simulink library "ddm"  (R2021b)
settings: Solver=VariableStepAuto  StartTime=0.0  StopTime=10.0  RelTol=1e-3
undefined symbols (not defined in the file or in its folder): ADDM_FrTMTqDev_X_Nm, ADDM_RrTMTqDev_X_Nm, ENUM_ADASACCSTA_ERROR, ENUM_ADASACCSTA_OFF, ENUM_ADASACCSTA_STANDBY, ENUM_ALLOWMOV_ALLOWREADY, ENUM_APS, ENUM_BRKSTA_ERROR, ENUM_BRKSTA_OFF, ENUM_BRKSTA_ON, ENUM_BRKSW_INVALID, ENUM_BRKSW_OFF, ENUM_BRKSW_ON, ENUM_CHGPREACTERRSTA_OBCPRE, ENUM_DCDCFAULTSTA_ANYFAULTLV1, ENUM_DCDCFAULTSTA_ANYFAULTLV2, ENUM_DRIVETRAIN_AWD, ENUM_DRIVETRAIN_FWD, ENUM_DRIVETRAIN_RWD, ENUM_EDUDRTSTA_NORMAL, ENUM_EPBSTA_APPLIED, ENUM_EPBSTA_RELEASED, ENUM_GEARACTUALPOSN_INVALID, ENUM_GEARACTUALPOSN_P, ENUM_HVBATTREADYPRE_READY, ENUM_MCUWARN_LV0, ENUM_MCUWARN_LV1, ENUM_MCUWARN_LV2, ENUM_MCUWARN_LV3, ENUM_MCUWARN_NOERROR, ENUM_OBCFAULTSTA_ANYFAULT, ENUM_PAS_R2F2, ENUM_PDFAULT_BATTPDFAIL, ENUM_PDFAULT_DCDCDISABLE, ENUM_PDFAULT_MCUDISABLE, ENUM_PDFAULT_MCUDISCHRG, ENUM_POWERSTA_OFF, ENUM_POWERSTA_ON, ENUM_POWERSTA_READY, ENUM_POWERSTA_STANDBY, ENUM_PRESSINDI_LOW, ENUM_PUFAULT_BATTUPFAIL, ENUM_PUFAULT_DCDCENABLEFAIL, ENUM_PUFAULT_PRECHRGCHKFAIL, ENUM_PUFAULT_SAFETYCHKFAIL, ENUM_PUSTATE_COMPLETED, ENUM_PWRSTASW_OFF, ENUM_PWRSTASW_OFFA, ENUM_PWRSTASW_OFFCHVCHRG, ENUM_PWRSTASW_OFFCLVCHRG, ENUM_PWRSTASW_ON, ENUM_PWRSTASW_ONHVCHRG, ENUM_PWRSTASW_READY, ENUM_PWRSTASW_STANDBY, ENUM_SHIFTCOMMAND_P, ENUM_SHIFTERERRSTA_PBUTTONFAILURE, ENUM_VEHMALFUNLV_2ND, ENUM_VEHMALFUNLV_3RD, ENUM_VEHMALFUNLV_4TH, ENUM_VEHMALFUNLV_NORMAL ... (+459)
libraries: hcu_lib x521, $bdroot x5, simulink x3
(part 14 of 25)

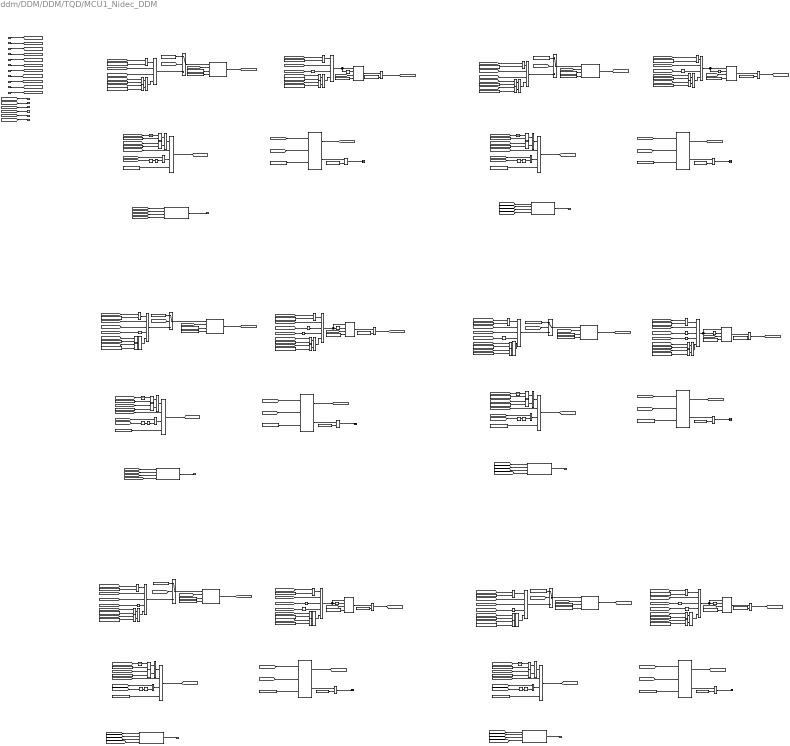
== system ddm/DDM/DDM/TQD/MCU1_Nidec_DDM ==
  note: Diagnostics and Fault Handling
  note: Release Condition After Decision
  note: Diagnostics and Fault Handling
  note: Release Condition After Decision
  note: Diagnostics and Fault Handling
  note: Release Condition After Decision
  note: Release Condition After Decision
  note: Diagnostics and Fault Handling
  note: Release Condition After Decision
  note: Diagnostics and Fault Handling
  note: Release Condition After Decision
  note: Diagnostics and Fault Handling
  note: MCU_F1 Lost Comm (MCUF1NoCom)
  note: MCU_R1 Lost Comm (MCUR1NoCom)
  note: MCU_R1 Rolling Count Error (MCUR1RCErr)
  note: MCU_F1 Rolling Count Error (MCUF1RCErr)
  note: MCU_R1 Checksum Error (MCUR1CSErr)
  note: MCU_F1 Checksum Error (MCUF1CSErr)
  task_time_s : Inport
  VPMM_SysPwrSta_enum : Inport  Port=2
  No_CAN3_BUS_OFF : Inport  Port=3
  VDDM_MCUNF1NoCom_flg : Inport  Port=4
  VDDM_MCUNR1NoCom_flg : Inport  Port=5
  VDDM_MCUNF1RCErr_flg : Inport  Port=6
  VDDM_MCUNF1CSErr_flg : Inport  Port=7
  VDDM_MCUNR1RCErr_flg : Inport  Port=8
  VDDM_MCUNR1CSErr_flg : Inport  Port=9
  DTC_clear_request : Inport  Port=10
  VPMM_DrivetrainSelect_enum : Inport  Port=11
  Constant{1..2,6..7,9,13,26,40,43,46,53,59..60,62,72,75,79,86} (18 alike) : Constant  Value=ENUM_PWRSTASW_OFF
  Constant{3,10,35,41,52,57} (6 alike) : Constant  Value=ENUM_PWRSTASW_STANDBY
  Constant{20,24,28,44,67,88,90,92,94,96,98,100} (12 alike) : Constant  Value=ENUM_DRIVETRAIN_AWD
  Constant{4,11,29,45,55,101} (6 alike) : Constant  Value=KDDM_TQDDiagnosisOffSW_flg
  Constant{5,12,30,49,56,102} (6 alike) : Constant  Value=ZERO_INT
  Constant14 : Constant  Value=KDDM_MCUF1NoComDTC_cnt
  Constant{15,27,66,93,95,97} (6 alike) : Constant  Value=ENUM_DRIVETRAIN_RWD
  Constant16 : Constant  Value=KDDM_MCUNR1NoComDTC_cnt
  Constant17 : Constant  Value=KDDM_MCUNR1NoComPassTO_s
  Constant18 : Constant  Value=KDDM_MCUNR1NoComPassTO_s
  Constant19 : Constant  Value=KDDM_MCUNR1NoComDetTO_s
  Constant{21,42,87,89,91,99} (6 alike) : Constant  Value=ENUM_DRIVETRAIN_FWD
  Constant{22..23,38..39,73..74} (6 alike) : Constant  Value=FALSE
  Constant25 : Constant  Value=KDDM_MCUF1RCErrDTC_cnt
  Constant31 : Constant  Value=KDDM_MCUNR1RCErrDTC_cnt
  Constant32 : Constant  Value=KDDM_MCUNR1RCErrPassTO_s
  Constant33 : Constant  Value=KDDM_MCUNR1RCErrPassTO_s
  Constant34 : Constant  Value=KDDM_MCUNR1RCErrDetTO_s
  Constant36 : Constant  Value=KDDM_MCUR1RCErrDTC_cnt
  Constant37 : Constant  Value=KDDM_MCUNF1CSErrPassTO_s
  Constant47 : Constant  Value=KDDM_MCUNF1RCErrDTC_cnt
  Constant48 : Constant  Value=KDDM_MCUNF1RCErrPassTO_s
  Constant50 : Constant  Value=KDDM_MCUNF1RCErrPassTO_s
  Constant51 : Constant  Value=KDDM_MCUNF1RCErrDetTO_s
  Constant54 : Constant  Value=KDDM_MCUF1RCErrDTC_cnt
  Constant58 : Constant  Value=KDDM_MCUR1RCErrDTC_cnt
  Constant61 : Constant  Value=KDDM_MCUNR1CSErrDTC_cnt
  Constant63 : Constant  Value=KDDM_MCUNR1CSErrPassTO_s
  Constant64 : Constant  Value=KDDM_MCUNR1CSErrPassTO_s
  Constant65 : Constant  Value=KDDM_MCUNR1CSErrDetTO_s
  Constant68 : Constant  Value=KDDM_MCUNF1NoComDTC_cnt
  Constant69 : Constant  Value=KDDM_MCUNF1NoComPassTO_s
  Constant70 : Constant  Value=KDDM_MCUNF1NoComPassTO_s
  Constant71 : Constant  Value=KDDM_MCUNF1NoComDetTO_s
  Constant8 : Constant  Value=KDDM_MCUR1NoComDTC_cnt
  Constant80 : Constant  Value=KDDM_MCUNF1CSErrDTC_cnt
  Constant83 : Constant  Value=KDDM_MCUNF1CSErrPassTO_s
  Constant84 : Constant  Value=KDDM_MCUNF1CSErrDetTO_s
  DTC_Couter{1..5,7} (6 alike) : hcu_lib/Basic_Blocks/DTC_Couter
  DTC_Info{,1..5} (6 alike) : hcu_lib/Basic_Blocks/DTC_Info
  Delay{1..6} (6 alike) : Delay  DelayLength=1
  Equal{,1..4,7..8,12,14..15,19..20,23,26..27,33..43,45,47..55} (36 alike) : RelationalOperator  Operator===  OutDataTypeStr=boolean  RndMeth=Simplest
  Equal{5,9..11,16,18,21..22,24,29,44,46} (12 alike) : RelationalOperator  Operator=~=  OutDataTypeStr=boolean  RndMeth=Simplest
  Equal{6,13,17,25,28,30} (6 alike) : RelationalOperator  OutDataTypeStr=boolean  RndMeth=Simplest
  Logical Operator{1,3,16,21,33,36} (6 alike) : Logic  Operator=OR  Inputs=4  AllPortsSameDT=off  OutDataTypeStr=boolean
  Logical Operator{6,10,13,15,19..20,24..26,29,32,37,41..42,61,70,81..84} (20 alike) : Logic  Operator=NOT  AllPortsSameDT=off  OutDataTypeStr=boolean
  Logical Operator{4,8..9,11,17..18,22,28,34..35,38..39} (12 alike) : Logic  AllPortsSameDT=off  OutDataTypeStr=boolean
  Logical Operator{7,12,23,27,31,40,58,67} (8 alike) : Logic  Inputs=5  AllPortsSameDT=off  OutDataTypeStr=boolean
  Logical Operator{2,5,14,30} (4 alike) : Logic  Inputs=4  AllPortsSameDT=off  OutDataTypeStr=boolean
  NOT{1..6} (6 alike) : Logic  Operator=NOT  AllPortsSameDT=off  OutDataTypeStr=boolean
  OR{,1..11} (12 alike) : Logic  Operator=OR  AllPortsSameDT=off  OutDataTypeStr=boolean
  Relational Operator{1..6} (6 alike) : RelationalOperator  Operator=>  OutDataTypeStr=boolean  RndMeth=Simplest
  Switch{1..6} (6 alike) : Switch  Criteria=u2 ~= 0
  Terminator{,1..5} (6 alike) : Terminator
  Test Detection Criteria{1..6} (6 alike) : hcu_lib/Basic_Blocks/Test Detection Criteria
  Timer{1..6} (6 alike) : hcu_lib/Basic_Blocks/Timer
  Unit Delay{1..4,6..7} (6 alike) : UnitDelay  SampleTime=-1  HasFrameUpgradeWarning=on
  VDDM_MCUF1NoComDTC_raw32 : Outport
  VDDM_MCUR1NoComDTC_raw32 : Outport  Port=2
  VDDM_MCUF1RCErrDTC_raw32 : Outport  Port=3
  VDDM_MCUR1RCErrDTC_raw32 : Outport  Port=4
  VDDM_MCUF1CSErrDTC_raw32 : Outport  Port=5
  VDDM_MCUR1CSErrDTC_raw32 : Outport  Port=6
  VDDM_MCUNF1NoComCFS_flg : Outport  Port=7
  VDDM_MCUNF1RCErrCFS_flg : Outport  Port=8
  VDDM_MCUNF1CSErrCFS_flg : Outport  Port=9
  VDDM_MCUNR1NoComCFS_flg : Outport  Port=10
  VDDM_MCUNR1RCErrCFS_flg : Outport  Port=11
  VDDM_MCUNR1CSErrCFS_flg : Outport  Port=12
  wires:
  Logical Operator42/1 -> Logical Operator40/3
  [VDDM_MCUNR1CSErr_flg] -> Logical Operator42/1
  [VPMM_DrivetrainSelect_enum] -> Equal54/1
  Logical Operator41/1 -> Logical Operator40/4
  Constant67/1 -> Equal55/2
  [VPMM_DrivetrainSelect_enum] -> Equal55/1
  Equal22/1 -> Logical Operator40/1
  Constant66/1 -> Equal54/2
  OR11/1 -> Logical Operator40/5
  Equal55/1 -> OR11/2
  [No_CAN3_BUS_OFF] -> Logical Operator40/2
  Constant60/1 -> Equal22/2
  [VDDM_MCUNR1NoComCFS_flg] -> Logical Operator41/1
  Equal54/1 -> OR11/1
  [VPMM_SysPwrSta_enum] -> Equal22/1
  [VPMM_SysPwrSta_enum] -> Unit Delay4/1
  NOT6/1 -> Logical Operator39/2
  [VDDM_MCUNR1CSErrPass_flg] -> Logical Operator39/1
  DTC_Couter5/2 -> Relational Operator6/1  "VDDM_MCUNR1CSErrDTC_cnt"
  Constant59/1 -> Equal27/2
  Relational Operator6/1 -> Terminator5/1  "VDDM_MCUNR1CSErrDFS_flg"
  Delay6/1 -> NOT6/1
  Unit Delay4/1 -> Equal27/1
  Constant58/1 -> DTC_Couter5/3
  Equal26/1 -> Logical Operator38/2
  Equal27/1 -> Logical Operator38/1
  [VPMM_SysPwrSta_enum] -> Equal26/1
  Logical Operator39/1 -> Logical Operator36/3
  Constant55/1 -> Logical Operator36/4
  Constant57/1 -> Equal26/2
  Logical Operator38/1 -> Logical Operator36/1
  Logical Operator36/1 -> [VDDM_MCUNR1CSErrCFSRls_flg]  "VDDM_MCUNR1CSErrCFSRls_flg"
  Constant56/1 -> Relational Operator6/2
  [VDDM_MCUNR1CSErrDet_flg] -> DTC_Couter5/1
  [DTC_clear_request] -> Logical Operator36/2
  [VDDM_MCUNR1CSErrCFS_flg] -> Delay6/1
  DTC_Couter5/1 -> [VDDM_MCUNR1CSErrCFS_flg]  "VDDM_MCUNR1CSErrCFS_flg"
  [VDDM_MCUNR1CSErrCFSRls_flg] -> DTC_Couter5/2
  [VPMM_SysPwrSta_enum] -> Equal52/1
  Constant75/1 -> Equal53/2
  [VDDM_MCUNF1CSErrDet_flg] -> DTC_Couter4/1
  Delay5/1 -> NOT5/1
  Unit Delay3/1 -> Equal53/1
  [VDDM_MCUNF1CSErrCFSRls_flg] -> DTC_Couter4/2
  Constant54/1 -> DTC_Couter4/3
  Equal53/1 -> Logical Operator34/1
  Equal52/1 -> Logical Operator34/2
  [VPMM_SysPwrSta_enum] -> Unit Delay3/1
  NOT5/1 -> Logical Operator35/2
  Logical Operator34/1 -> Logical Operator33/1
  Constant52/1 -> Equal52/2
  Constant45/1 -> Logical Operator33/4
  [DTC_clear_request] -> Logical Operator33/2
  Logical Operator35/1 -> Logical Operator33/3
  DTC_Couter4/2 -> Relational Operator5/1  "VDDM_MCUNF1CSErrDTC_cnt"
  [VDDM_MCUNF1CSErrPass_flg] -> Logical Operator35/1
  Logical Operator33/1 -> [VDDM_MCUNF1CSErrCFSRls_flg]  "VDDM_MCUNF1CSErrCFSRls_flg"
  Constant49/1 -> Relational Operator5/2
  Relational Operator5/1 -> Terminator4/1  "VDDM_MCUNF1CSErrDFS_flg"
  DTC_Couter4/1 -> [VDDM_MCUNF1CSErrCFS_flg]  "VDDM_MCUNF1CSErrCFS_flg"
  [VDDM_MCUNF1CSErrCFS_flg] -> Delay5/1
  Logical Operator32/1 -> Logical Operator27/3
  OR10/1 -> Logical Operator27/5
  Equal20/1 -> OR10/2
  Equal19/1 -> OR10/1
  [VPMM_DrivetrainSelect_enum] -> Equal19/1
  Constant42/1 -> Equal19/2
  Constant44/1 -> Equal20/2
  [VPMM_DrivetrainSelect_enum] -> Equal20/1
  [VDDM_MCUNF1NoComCFS_flg] -> Logical Operator29/1
  Logical Operator29/1 -> Logical Operator27/4
  [VDDM_MCUNF1CSErr_flg] -> Logical Operator32/1
  Constant40/1 -> Equal18/2
  Equal18/1 -> Logical Operator27/1
  [No_CAN3_BUS_OFF] -> Logical Operator27/2
  [VPMM_SysPwrSta_enum] -> Equal18/1
  Logical Operator6/1 -> Logical Operator5/3
  Logical Operator25/1 -> Timer2/2
  Logical Operator24/1 -> Logical Operator2/3
  Logical Operator10/1 -> Timer1/2
  [VPMM_SysPwrSta_enum] -> Equal15/1
  Constant43/1 -> Equal51/2
  [VDDM_MCUNR1RCErrDet_flg] -> DTC_Couter3/1
  Delay4/1 -> NOT4/1
  Unit Delay2/1 -> Equal51/1
  [VDDM_MCUNR1RCErrCFSRls_flg] -> DTC_Couter3/2
  Constant36/1 -> DTC_Couter3/3
  Equal51/1 -> Logical Operator22/1
  Equal15/1 -> Logical Operator22/2
  [VPMM_SysPwrSta_enum] -> Unit Delay2/1
  NOT4/1 -> Logical Operator28/2
  Logical Operator22/1 -> Logical Operator21/1
  Constant35/1 -> Equal15/2
  Constant29/1 -> Logical Operator21/4
  [DTC_clear_request] -> Logical Operator21/2
  Logical Operator28/1 -> Logical Operator21/3
  DTC_Couter3/2 -> Relational Operator4/1  "VDDM_MCUNR1RCErrDTC_cnt"
  [VDDM_MCUNR1RCErrPass_flg] -> Logical Operator28/1
  Logical Operator21/1 -> [VDDM_MCUNR1RCErrCFSRls_flg]  "VDDM_MCUNR1RCErrCFSRls_flg"
  Constant30/1 -> Relational Operator4/2
  Relational Operator4/1 -> Terminator3/1  "VDDM_MCUNR1RCErrDFS_flg"
  DTC_Couter3/1 -> [VDDM_MCUNR1RCErrCFS_flg]  "VDDM_MCUNR1RCErrCFS_flg"
  [VDDM_MCUNR1RCErrCFS_flg] -> Delay4/1
  Logical Operator20/1 -> Logical Operator7/3
  OR9/1 -> Logical Operator7/5
  [VPMM_DrivetrainSelect_enum] -> Equal14/1
  Constant27/1 -> Equal12/2
  Equal14/1 -> OR9/2
  [VPMM_DrivetrainSelect_enum] -> Equal12/1
  Constant28/1 -> Equal14/2
  Equal12/1 -> OR9/1
  [VDDM_MCUNR1NoComCFS_flg] -> Logical Operator19/1
  Logical Operator19/1 -> Logical Operator7/4
  [No_CAN3_BUS_OFF] -> Logical Operator7/2
  Equal10/1 -> Logical Operator7/1
  Constant26/1 -> Equal10/2
  [VDDM_MCUNR1RCErr_flg] -> Logical Operator20/1
  [VPMM_SysPwrSta_enum] -> Equal10/1
  Delay3/1 -> NOT3/1
  [VDDM_MCUNF1RCErrCFS_flg] -> Delay3/1
  Constant101/1 -> Logical Operator16/4
  [DTC_clear_request] -> Logical Operator16/2
  NOT3/1 -> Logical Operator18/2
  Constant41/1 -> Equal49/2
  Logical Operator17/1 -> Logical Operator16/1
  [VPMM_SysPwrSta_enum] -> Unit Delay7/1
  Relational Operator3/1 -> Terminator2/1  "VDDM_MCUNF1RCErrDFS_flg"
  Equal49/1 -> Logical Operator17/2
  Constant72/1 -> Equal50/2
  Unit Delay7/1 -> Equal50/1
  [VPMM_SysPwrSta_enum] -> Equal49/1
  Equal50/1 -> Logical Operator17/1
  [VDDM_MCUNF1RCErrPass_flg] -> Logical Operator18/1
  Logical Operator18/1 -> Logical Operator16/3
  Constant25/1 -> DTC_Couter7/3
  DTC_Couter7/1 -> [VDDM_MCUNF1RCErrCFS_flg]  "VDDM_MCUNF1RCErrCFS_flg"
  Logical Operator16/1 -> [VDDM_MCUNF1RCErrCFSRls_flg]  "VDDM_MCUNF1RCErrCFSRls_flg"
  [VDDM_MCUNF1RCErrCFSRls_flg] -> DTC_Couter7/2
  DTC_Couter7/2 -> Relational Operator3/1  "VDDM_MCUNF1RCErrDTC_cnt"
  [VDDM_MCUNF1RCErrDet_flg] -> DTC_Couter7/1
  Constant102/1 -> Relational Operator3/2
  Logical Operator15/1 -> Logical Operator12/3
  [VPMM_DrivetrainSelect_enum] -> Equal48/1
  Constant24/1 -> Equal48/2
  [VDDM_MCUNF1NoComCFS_flg] -> Logical Operator13/1
  Equal47/1 -> OR8/1
  [VPMM_SysPwrSta_enum] -> Equal9/1
  Logical Operator13/1 -> Logical Operator12/4
  Constant21/1 -> Equal47/2
  Equal9/1 -> Logical Operator12/1
  Equal48/1 -> OR8/2
  [VPMM_DrivetrainSelect_enum] -> Equal47/1
  OR8/1 -> Logical Operator12/5
  [VDDM_MCUNF1RCErr_flg] -> Logical Operator15/1
  Constant7/1 -> Equal9/2
  [No_CAN3_BUS_OFF] -> Logical Operator12/2
  Delay2/1 -> NOT2/1
  [VDDM_MCUNR1NoComCFS_flg] -> Delay2/1
  Constant4/1 -> Logical Operator1/4
  [DTC_clear_request] -> Logical Operator1/2
  NOT2/1 -> Logical Operator11/2
  Constant3/1 -> Equal7/2
  Logical Operator9/1 -> Logical Operator1/1
  [VPMM_SysPwrSta_enum] -> Unit Delay1/1
  Relational Operator1/1 -> Terminator1/1  "VDDM_MCUNR1NoComDFS_flg"
  Equal7/1 -> Logical Operator9/2
  Constant6/1 -> Equal8/2
  Unit Delay1/1 -> Equal8/1
  [VPMM_SysPwrSta_enum] -> Equal7/1
  Equal8/1 -> Logical Operator9/1
  [VDDM_MCUNR1NoComPass_flg] -> Logical Operator11/1
  Logical Operator11/1 -> Logical Operator1/3
  Constant8/1 -> DTC_Couter2/3
  DTC_Couter2/1 -> [VDDM_MCUNR1NoComCFS_flg]  "VDDM_MCUNR1NoComCFS_flg"
  Logical Operator1/1 -> [VDDM_MCUNR1NoComCFSRls_flg]  "VDDM_MCUNR1NoComCFSRls_flg"
  [VDDM_MCUNR1NoComCFSRls_flg] -> DTC_Couter2/2
  DTC_Couter2/2 -> Relational Operator1/1  "VDDM_MCUNR1NoComDTC_cnt"
  [VDDM_MCUNR1NoComDet_flg] -> DTC_Couter2/1
  Constant5/1 -> Relational Operator1/2
  Logical Operator5/1 -> Logical Operator25/1, Timer2/1
  Equal2/1 -> OR7/1
  Constant20/1 -> Equal23/2
  OR7/1 -> Logical Operator5/4
  [VPMM_DrivetrainSelect_enum] -> Equal2/1
  Equal23/1 -> OR7/2
  Constant15/1 -> Equal2/2
  [VPMM_DrivetrainSelect_enum] -> Equal23/1
  [No_CAN3_BUS_OFF] -> Logical Operator5/2
  Constant2/1 -> Equal46/2
  [VDDM_MCUNR1NoCom_flg] -> Logical Operator6/1
  Equal46/1 -> Logical Operator5/1
  [VPMM_SysPwrSta_enum] -> Equal46/1
  Constant13/1 -> Equal4/2
  [VPMM_SysPwrSta_enum] -> Equal3/1
  Constant10/1 -> Equal3/2
  Equal4/1 -> Logical Operator4/1
  [DTC_clear_request] -> Logical Operator3/2
  Logical Operator8/1 -> Logical Operator3/3
  Logical Operator4/1 -> Logical Operator3/1
  [VDDM_MCUNF1NoComPass_flg] -> Logical Operator8/1
  Constant11/1 -> Logical Operator3/4
  Logical Operator3/1 -> [VDDM_MCUNF1NoComCFSRls_flg]  "VDDM_MCUNF1NoComCFSRls_flg"
  NOT1/1 -> Logical Operator8/2
  [VDDM_MCUNF1NoComCFS_flg] -> Delay1/1
  Delay1/1 -> NOT1/1
  Equal3/1 -> Logical Operator4/2
  Unit Delay6/1 -> Equal4/1
  [VPMM_SysPwrSta_enum] -> Unit Delay6/1
  DTC_Couter1/2 -> Relational Operator2/1  "VDDM_MCUNF1NoComDTC_cnt"
  Relational Operator2/1 -> Terminator/1  "VDDM_MCUNF1NoComDFS_flg"
  Constant12/1 -> Relational Operator2/2
  Logical Operator2/1 -> Logical Operator10/1, Timer1/1
  [VPMM_SysPwrSta_enum] -> Equal44/1
  Equal1/1 -> OR6/1
  [VDDM_MCUNF1NoCom_flg] -> Logical Operator24/1
  Constant99/1 -> Equal1/2
  Equal44/1 -> Logical Operator2/1
  Constant100/1 -> Equal45/2
  [No_CAN3_BUS_OFF] -> Logical Operator2/2
  [VPMM_DrivetrainSelect_enum] -> Equal45/1
  OR6/1 -> Logical Operator2/4
  Equal45/1 -> OR6/2
  Constant1/1 -> Equal44/2
  [VPMM_DrivetrainSelect_enum] -> Equal1/1
  [VDDM_MCUNF1NoCom_flg] -> Logical Operator30/3
  Equal21/1 -> Logical Operator30/1
  [No_CAN3_BUS_OFF] -> Logical Operator30/2
  Timer1/1 -> Equal28/1
  [VDDM_MCUNF1NoComDet_flg] -> DTC_Couter1/1
  [VPMM_SysPwrSta_enum] -> Equal21/1
  Constant70/1 -> Timer1/4
  [task_time_s] -> Timer1/3
  Test Detection Criteria1/1 -> [VDDM_MCUNF1NoComDet_flg]  "VDDM_MCUNF1NoComDet_flg"
  Constant62/1 -> Equal21/2
  Constant69/1 -> Equal28/2
  Equal28/1 -> [VDDM_MCUNF1NoComPass_flg]  "VDDM_MCUNF1NoComPass_flg"
  [task_time_s] -> Test Detection Criteria1/2
  Constant68/1 -> Test Detection Criteria1/3
  Constant71/1 -> Test Detection Criteria1/4
  Constant14/1 -> DTC_Couter1/3
  [VDDM_MCUNF1NoComCFSRls_flg] -> DTC_Couter1/2
  [VPMM_SysPwrSta_enum] -> Equal5/1
  Equal5/1 -> Logical Operator14/1
  Constant19/1 -> Test Detection Criteria2/4
  Timer2/1 -> Equal6/1
  Equal6/1 -> [VDDM_MCUNR1NoComPass_flg]  "VDDM_MCUNR1NoComPass_flg"
  Test Detection Criteria2/1 -> [VDDM_MCUNR1NoComDet_flg]  "VDDM_MCUNR1NoComDet_flg"
  Constant16/1 -> Test Detection Criteria2/3
  [VDDM_MCUNR1NoCom_flg] -> Logical Operator14/3
  Constant18/1 -> Timer2/4
  Constant9/1 -> Equal5/2
  [No_CAN3_BUS_OFF] -> Logical Operator14/2
  [task_time_s] -> Test Detection Criteria2/2
  Constant17/1 -> Equal6/2
  [task_time_s] -> Timer2/3
  [VDDM_MCUNF1NoComCFS_flg] -> DTC_Info/3
  [VDDM_MCUNF1NoComPass_flg] -> DTC_Info/2
  [VDDM_MCUNF1NoComDet_flg] -> DTC_Info/1
  DTC_Info/1 -> VDDM_MCUF1NoComDTC_raw32/1  "VDDM_MCUF1NoComDTC_raw32"
  [VDDM_MCUNR1NoComDet_flg] -> DTC_Info1/1
  DTC_Info1/1 -> VDDM_MCUR1NoComDTC_raw32/1  "VDDM_MCUR1NoComDTC_raw32"
  [VDDM_MCUNR1NoComCFS_flg] -> DTC_Info1/3
  [VDDM_MCUNR1NoComPass_flg] -> DTC_Info1/2
  task_time_s/1 -> [task_time_s]
  VPMM_SysPwrSta_enum/1 -> [VPMM_SysPwrSta_enum]
  No_CAN3_BUS_OFF/1 -> [No_CAN3_BUS_OFF]
  VDDM_MCUNF1NoCom_flg/1 -> [VDDM_MCUNF1NoCom_flg]
  DTC_clear_request/1 -> [DTC_clear_request]
  VDDM_MCUNR1NoCom_flg/1 -> [VDDM_MCUNR1NoCom_flg]
  DTC_Couter1/1 -> [VDDM_MCUNF1NoComCFS_flg]  "VDDM_MCUNF1NoComCFS_flg"
  [DTC_clear_request] -> DTC_Info/4
  [DTC_clear_request] -> DTC_Info1/4
  [VDDM_MCUNF1NoComCFSRls_flg] -> Switch6/2
  Switch6/1 -> Test Detection Criteria1/1
  Constant22/1 -> Switch6/1
  Logical Operator30/1 -> Switch6/3
  [VDDM_MCUNR1NoComCFSRls_flg] -> Switch1/2
  Switch1/1 -> Test Detection Criteria2/1
  Constant23/1 -> Switch1/1
  [VPMM_SysPwrSta_enum] -> Equal11/1
  [No_CAN3_BUS_OFF] -> Logical Operator31/2
  Logical Operator37/1 -> Timer3/2
  [VPMM_SysPwrSta_enum] -> Equal16/1
  Timer3/1 -> Equal13/1
  Constant48/1 -> Equal13/2
  Logical Operator7/1 -> Timer4/1, Logical Operator26/1
  Test Detection Criteria3/1 -> [VDDM_MCUNF1RCErrDet_flg]  "VDDM_MCUNF1RCErrDet_flg"
  Constant51/1 -> Test Detection Criteria3/4
  Equal11/1 -> Logical Operator31/1
  Constant50/1 -> Timer3/4
  Constant34/1 -> Test Detection Criteria4/4
  Constant46/1 -> Equal11/2
  Equal17/1 -> [VDDM_MCUNR1RCErrPass_flg]  "VDDM_MCUNR1RCErrPass_flg"
  [VDDM_MCUNF1RCErr_flg] -> Logical Operator31/3
  Test Detection Criteria4/1 -> [VDDM_MCUNR1RCErrDet_flg]  "VDDM_MCUNR1RCErrDet_flg"
  DTC_Info2/1 -> VDDM_MCUF1RCErrDTC_raw32/1  "VDDM_MCUF1RCErrDTC_raw32"
  [VDDM_MCUNF1RCErrDet_flg] -> DTC_Info2/1
  [VDDM_MCUNF1RCErrPass_flg] -> DTC_Info2/2
  DTC_Info3/1 -> VDDM_MCUR1RCErrDTC_raw32/1  "VDDM_MCUR1RCErrDTC_raw32"
  [task_time_s] -> Timer4/3
  [task_time_s] -> Test Detection Criteria3/2
  [VDDM_MCUNR1RCErrPass_flg] -> DTC_Info3/2
  Timer4/1 -> Equal17/1
  [VDDM_MCUNR1RCErrDet_flg] -> DTC_Info3/1
  [VDDM_MCUNR1RCErr_flg] -> Logical Operator23/3
  Constant33/1 -> Timer4/4
  [VDDM_MCUNF1RCErrCFSRls_flg] -> Switch3/2
  Constant53/1 -> Equal16/2
  Constant47/1 -> Test Detection Criteria3/3
  [task_time_s] -> Timer3/3
  Equal13/1 -> [VDDM_MCUNF1RCErrPass_flg]  "VDDM_MCUNF1RCErrPass_flg"
  Equal16/1 -> Logical Operator23/1
  [VDDM_MCUNR1RCErrCFS_flg] -> DTC_Info3/3
  Logical Operator12/1 -> Timer3/1, Logical Operator37/1
  Constant32/1 -> Equal17/2
  [VDDM_MCUNF1RCErrCFS_flg] -> DTC_Info2/3
  Constant38/1 -> Switch3/1
  [No_CAN3_BUS_OFF] -> Logical Operator23/2
  Switch3/1 -> Test Detection Criteria3/1
  Logical Operator26/1 -> Timer4/2
  Constant31/1 -> Test Detection Criteria4/3
  [VDDM_MCUNR1RCErrCFSRls_flg] -> Switch2/2
  [task_time_s] -> Test Detection Criteria4/2
  Switch2/1 -> Test Detection Criteria4/1
  Constant39/1 -> Switch2/1
  [DTC_clear_request] -> DTC_Info2/4
  [DTC_clear_request] -> DTC_Info3/4
  [VPMM_SysPwrSta_enum] -> Equal24/1
  [No_CAN3_BUS_OFF] -> Logical Operator67/2
  Logical Operator70/1 -> Timer5/2
  [VPMM_SysPwrSta_enum] -> Equal29/1
  Timer5/1 -> Equal25/1
  Constant37/1 -> Equal25/2
  Logical Operator40/1 -> Logical Operator61/1, Timer6/1
  Test Detection Criteria5/1 -> [VDDM_MCUNF1CSErrDet_flg]  "VDDM_MCUNF1CSErrDet_flg"
  Constant84/1 -> Test Detection Criteria5/4
  Equal24/1 -> Logical Operator67/1
  Constant83/1 -> Timer5/4
  Constant65/1 -> Test Detection Criteria6/4
  Constant79/1 -> Equal24/2
  Equal30/1 -> [VDDM_MCUNR1CSErrPass_flg]  "VDDM_MCUNR1CSErrPass_flg"
  [VDDM_MCUNF1CSErr_flg] -> Logical Operator67/3
  Test Detection Criteria6/1 -> [VDDM_MCUNR1CSErrDet_flg]  "VDDM_MCUNR1CSErrDet_flg"
  DTC_Info4/1 -> VDDM_MCUF1CSErrDTC_raw32/1  "VDDM_MCUF1CSErrDTC_raw32"
  [VDDM_MCUNF1CSErrDet_flg] -> DTC_Info4/1
  [VDDM_MCUNF1CSErrPass_flg] -> DTC_Info4/2
  DTC_Info5/1 -> VDDM_MCUR1CSErrDTC_raw32/1  "VDDM_MCUR1CSErrDTC_raw32"
  [task_time_s] -> Timer6/3
  [task_time_s] -> Test Detection Criteria5/2
  [VDDM_MCUNR1CSErrPass_flg] -> DTC_Info5/2
  Timer6/1 -> Equal30/1
  [VDDM_MCUNR1CSErrDet_flg] -> DTC_Info5/1
  [VDDM_MCUNR1CSErr_flg] -> Logical Operator58/3
  Constant64/1 -> Timer6/4
  [VDDM_MCUNF1CSErrCFSRls_flg] -> Switch5/2
  Constant86/1 -> Equal29/2
  Constant80/1 -> Test Detection Criteria5/3
  [task_time_s] -> Timer5/3
  Equal25/1 -> [VDDM_MCUNF1CSErrPass_flg]  "VDDM_MCUNF1CSErrPass_flg"
  Equal29/1 -> Logical Operator58/1
  [VDDM_MCUNR1CSErrCFS_flg] -> DTC_Info5/3
  Logical Operator27/1 -> Logical Operator70/1, Timer5/1
  Constant63/1 -> Equal30/2
  [VDDM_MCUNF1CSErrCFS_flg] -> DTC_Info4/3
  Constant73/1 -> Switch5/1
  [No_CAN3_BUS_OFF] -> Logical Operator58/2
  Switch5/1 -> Test Detection Criteria5/1
  Logical Operator61/1 -> Timer6/2
  Constant61/1 -> Test Detection Criteria6/3
  [VDDM_MCUNR1CSErrCFSRls_flg] -> Switch4/2
  [task_time_s] -> Test Detection Criteria6/2
  Switch4/1 -> Test Detection Criteria6/1
  Constant74/1 -> Switch4/1
  [DTC_clear_request] -> DTC_Info4/4
  [DTC_clear_request] -> DTC_Info5/4
  [VDDM_MCUNF1NoComCFS_flg] -> Logical Operator81/1
  Logical Operator81/1 -> Logical Operator31/4
  Logical Operator82/1 -> Logical Operator23/4
  [VDDM_MCUNR1NoComCFS_flg] -> Logical Operator82/1
  Logical Operator83/1 -> Logical Operator67/4
  [VDDM_MCUNF1NoComCFS_flg] -> Logical Operator83/1
  Logical Operator84/1 -> Logical Operator58/4
  [VDDM_MCUNR1NoComCFS_flg] -> Logical Operator84/1
  VDDM_MCUNF1RCErr_flg/1 -> [VDDM_MCUNF1RCErr_flg]
  VDDM_MCUNF1CSErr_flg/1 -> [VDDM_MCUNF1CSErr_flg]
  VDDM_MCUNR1RCErr_flg/1 -> [VDDM_MCUNR1RCErr_flg]
  VDDM_MCUNR1CSErr_flg/1 -> [VDDM_MCUNR1CSErr_flg]
  Logical Operator31/1 -> Switch3/3
  Logical Operator67/1 -> Switch5/3
  Logical Operator14/1 -> Switch1/3
  Logical Operator23/1 -> Switch2/3
  Logical Operator58/1 -> Switch4/3
  [VDDM_MCUNF1NoComCFS_flg] -> VDDM_MCUNF1NoComCFS_flg/1
  [VDDM_MCUNF1CSErrCFS_flg] -> VDDM_MCUNF1CSErrCFS_flg/1
  [VDDM_MCUNR1CSErrCFS_flg] -> VDDM_MCUNR1CSErrCFS_flg/1
  [VDDM_MCUNR1RCErrCFS_flg] -> VDDM_MCUNR1RCErrCFS_flg/1
  [VDDM_MCUNR1NoComCFS_flg] -> VDDM_MCUNR1NoComCFS_flg/1
  [VDDM_MCUNF1RCErrCFS_flg] -> VDDM_MCUNF1RCErrCFS_flg/1
  VPMM_DrivetrainSelect_enum/1 -> [VPMM_DrivetrainSelect_enum]
  Equal/1 -> OR/1
  Equal33/1 -> OR/2
  Constant87/1 -> Equal/2
  [VPMM_DrivetrainSelect_enum] -> Equal33/1
  Constant88/1 -> Equal33/2
  OR/1 -> Logical Operator30/4
  [VPMM_DrivetrainSelect_enum] -> Equal35/1
  Constant89/1 -> Equal34/2
  Equal35/1 -> OR1/2
  [VPMM_DrivetrainSelect_enum] -> Equal34/1
  OR1/1 -> Logical Operator31/5
  Constant90/1 -> Equal35/2
  Equal34/1 -> OR1/1
  [VPMM_DrivetrainSelect_enum] -> Equal37/1
  Constant92/1 -> Equal37/2
  Constant91/1 -> Equal36/2
  [VPMM_DrivetrainSelect_enum] -> Equal36/1
  Equal36/1 -> OR2/1
  Equal37/1 -> OR2/2
  OR2/1 -> Logical Operator67/5
  [VPMM_DrivetrainSelect_enum] -> Equal39/1
  Constant93/1 -> Equal38/2
  Equal39/1 -> OR3/2
  [VPMM_DrivetrainSelect_enum] -> Equal38/1
  OR3/1 -> Logical Operator14/4
  Constant94/1 -> Equal39/2
  Equal38/1 -> OR3/1
  Equal40/1 -> OR4/1
  Constant96/1 -> Equal41/2
  [VPMM_DrivetrainSelect_enum] -> Equal40/1
  Equal41/1 -> OR4/2
  Constant95/1 -> Equal40/2
  [VPMM_DrivetrainSelect_enum] -> Equal41/1
  OR4/1 -> Logical Operator23/5
  Constant97/1 -> Equal42/2
  [VPMM_DrivetrainSelect_enum] -> Equal43/1
  [VPMM_DrivetrainSelect_enum] -> Equal42/1
  Constant98/1 -> Equal43/2
  Equal42/1 -> OR5/1
  Equal43/1 -> OR5/2
  OR5/1 -> Logical Operator58/5
  [VPMM_DrivetrainSelect_enum] -> Equal/1

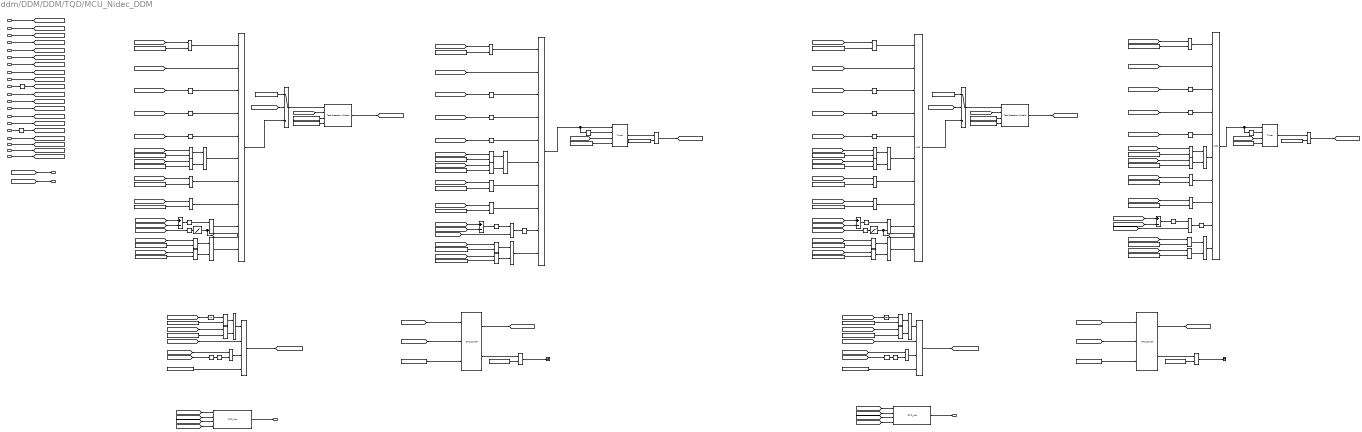
== system ddm/DDM/DDM/TQD/MCU_Nidec_DDM ==
  note: VINP_FrEDUDrtStaNidec_flg
  note: Front Motor Torque Response Error (FrMCUTqErr)
  note: Test Pass Creteria
  note: Test Dtection Criteria
  note: Test Pass Creteria
  note: Rear Motor Torque Response Error (RrMCUTqErr)
  note: Test Dtection Criteria
  note: Diagnostics and Fault Handling
  note: Release Condition After Decision
  note: Release Condition After Decision
  note: Diagnostics and Fault Handling
  task_time_s : Inport
  VPMM_SysPwrSta_enum : Inport  Port=2
  No_CAN3_BUS_OFF : Inport  Port=3
  VDDM_MCUNF1NoComCFS_flg : Inport  Port=4
  VDDM_MCUNF1RCErrCFS_flg : Inport  Port=5
  VDDM_MCUNF1CSErrCFS_flg : Inport  Port=6
  VINP_VehSpeed_kph : Inport  Port=7
  VINP_FrEDUDrtStaNidec_flg : Inport  Port=8
  VINP_FrEDURealTMTqNidec_Nm : Inport  Port=9
  VTQR_FrTMTqReq_Nm : Inport  Port=10
  VDDM_MCUNR1NoComCFS_flg : Inport  Port=11
  VDDM_MCUNR1RCErrCFS_flg : Inport  Port=12
  VDDM_MCUNR1CSErrCFS_flg : Inport  Port=13
  VINP_RrEDUDrtStaNidec_flg : Inport  Port=14
  VINP_RrEDURealTMTqNidec_Nm : Inport  Port=15
  VTQR_RrTMTqReq_Nm : Inport  Port=16
  VINP_MCUWarnFNidec_enum : Inport  Port=17
  VINP_MCUWarnRNidec_enum : Inport  Port=18
  DTC_clear_request : Inport  Port=19
  VPMM_DrivetrainSelect_enum : Inport  Port=20
  Abs{,1..4,6} (6 alike) : Abs
  Add{,1..3} (4 alike) : Sum  Inputs=+-
  Constant1 : Constant  Value=ENUM_DRIVETRAIN_FWD
  Constant10 : Constant  Value=KDDM_RrMCUNTqErrSpd_kph
  Constant{4,11,16,32} (4 alike) : Constant  Value=ENUM_MCUWARN_LV0
  Constant12 : Constant  Value=ENUM_PWRSTASW_STANDBY
  Constant{13,17,19,23,33,44} (6 alike) : Constant  Value=ENUM_PWRSTASW_OFF
  Constant{5,14,21,34} (4 alike) : Constant  Value=ENUM_MCUWARN_NOERROR
  Constant15 : Constant  Value=ENUM_DRIVETRAIN_FWD
  Constant18 : Constant  Value=KDDM_RrMCUTqErrDTC_cnt
  Constant2 : Constant  Value=ENUM_DRIVETRAIN_RWD
  Constant{8,20,26,49} (4 alike) : Constant  Value=ENUM_DRIVETRAIN_AWD
  Constant22 : Constant  Value=ENUM_PWRSTASW_STANDBY
  Constant24 : Constant  Value=FALSE
  Constant{6,25,35,41} (4 alike) : Constant  Value=ENUM_EDUDRTSTA_NORMAL
  Constant28 : Constant  Value=KDDM_RrMCUNTqErrDTC_cnt
  Constant29 : Constant  Value=KDDM_TQDDiagnosisOffSW_flg
  Constant3 : Constant  Value=KDDM_FrMCUNTqErrSpd_kph
  Constant30 : Constant  Value=ZERO_INT
  Constant31 : Constant  Value=KDDM_RrMCUNTqErrSpd_kph
  Constant36 : Constant  Value=KDDM_RrMCUNTqErrPassTO_s
  Constant37 : Constant  Value=KDDM_RrMCUNTqErrDetTO_s
  Constant39 : Constant  Value=KDDM_RrMCUNTqErrPassTO_s
  Constant42 : Constant  Value=FALSE
  Constant43 : Constant  Value=KDDM_FrMCUNTqErrDTC_cnt
  Constant45 : Constant  Value=KDDM_FrMCUNTqErrPassTO_s
  Constant46 : Constant  Value=KDDM_FrMCUNTqErrDetTO_s
  Constant51 : Constant  Value=KDDM_TQDDiagnosisOffSW_flg
  Constant52 : Constant  Value=ZERO_INT
  Constant54 : Constant  Value=KDDM_FrMCUTqErrDTC_cnt
  Constant7 : Constant  Value=KDDM_FrMCUNTqErrSpd_kph
  Constant70 : Constant  Value=KDDM_FrMCUNTqErrPassTO_s
  Constant9 : Constant  Value=ENUM_DRIVETRAIN_RWD
  DTC_Couter1 : hcu_lib/Basic_Blocks/DTC_Couter
  DTC_Couter3 : hcu_lib/Basic_Blocks/DTC_Couter
  DTC_Info : hcu_lib/Basic_Blocks/DTC_Info
  DTC_Info1 : hcu_lib/Basic_Blocks/DTC_Info
  Delay1 : Delay  DelayLength=1
  Delay2 : Delay  DelayLength=1
  Equal{,1,3..4,6..7,9..11,15,20..22,25,28..37} (24 alike) : RelationalOperator  Operator===  OutDataTypeStr=boolean  RndMeth=Simplest
  Equal{5,8,12..13,18,27} (6 alike) : RelationalOperator  OutDataTypeStr=boolean  RndMeth=Simplest
  Equal{2,14,17,23} (4 alike) : RelationalOperator  Operator=>  OutDataTypeStr=boolean  RndMeth=Simplest
  Equal{16,19,24,26} (4 alike) : RelationalOperator  Operator=~=  OutDataTypeStr=boolean  RndMeth=Simplest
  Logical Operator{1..2,4,16} (4 alike) : Logic  Operator=OR  AllPortsSameDT=off  OutDataTypeStr=boolean
  Logical Operator{3,5,7..10,12..15,17..18,28,34..35,37} (16 alike) : Logic  Operator=NOT  AllPortsSameDT=off  OutDataTypeStr=boolean
  Logical Operator{6,11,27,30} (4 alike) : Logic  Inputs=10  AllPortsSameDT=off  OutDataTypeStr=boolean
  Logical Operator19 : Logic  Operator=OR  Inputs=4  AllPortsSameDT=off  OutDataTypeStr=boolean
  Logical Operator{20..22,43} (4 alike) : Logic  AllPortsSameDT=off  OutDataTypeStr=boolean
  Logical Operator41 : Logic  Operator=OR  Inputs=4  AllPortsSameDT=off  OutDataTypeStr=boolean
  MDDM_FrTMTqDev_Y_Nm : Lookup_n-D  NumberOfTableDimensions=1  BreakpointsForDimension1=ADDM_FrTMTqDev_X_Nm  Table=MDDM_FrTMTqDev_Y_Nm  InternalRulePriority=Speed  RndMeth=Simplest  InputSameDT=on
  MDDM_RrTMTqDev_Y_Nm : Lookup_n-D  NumberOfTableDimensions=1  BreakpointsForDimension1=ADDM_RrTMTqDev_X_Nm  Table=MDDM_RrTMTqDev_Y_Nm  InternalRulePriority=Speed  RndMeth=Simplest  InputSameDT=on
  NOT1 : Logic  Operator=NOT  AllPortsSameDT=off  OutDataTypeStr=boolean
  NOT2 : Logic  Operator=NOT  AllPortsSameDT=off  OutDataTypeStr=boolean
  OR{,1..3} (4 alike) : Logic  Operator=OR  AllPortsSameDT=off  OutDataTypeStr=boolean
  Relational Operator1 : RelationalOperator  Operator=>  OutDataTypeStr=boolean  RndMeth=Simplest
  Relational Operator2 : RelationalOperator  Operator=>  OutDataTypeStr=boolean  RndMeth=Simplest
  Round : Rounding  Operator=round
  Round1 : Rounding  Operator=round
  Switch1 : Switch  Criteria=u2 ~= 0
  Switch6 : Switch  Criteria=u2 ~= 0
  Terminator : Terminator
  Terminator1 : Terminator
  Test Detection Criteria1 : hcu_lib/Basic_Blocks/Test Detection Criteria
  Test Detection Criteria2 : hcu_lib/Basic_Blocks/Test Detection Criteria
  Timer1 : hcu_lib/Basic_Blocks/Timer
  Timer2 : hcu_lib/Basic_Blocks/Timer
  Unit Delay1 : UnitDelay  SampleTime=-1  HasFrameUpgradeWarning=on
  Unit Delay5 : UnitDelay  SampleTime=-1  HasFrameUpgradeWarning=on
  VDDM_FrMCUTqErrDTC_raw32 : Outport
  VDDM_RrMCUTqErrDTC_raw32 : Outport  Port=2
  VDDM_FrMCUNTqErrCFS_flg : Outport  Port=3
  VDDM_RrMCUNTqErrCFS_flg : Outport  Port=4
  wires:
  Equal26/1 -> Logical Operator30/1
  Constant44/1 -> Equal26/2
  [VPMM_SysPwrSta_enum] -> Equal26/1
  [No_CAN_BUS_OFF] -> Logical Operator30/2
  Constant3/1 -> Equal2/2
  [VINP_VehSpeed_kph] -> Equal2/1
  Constant4/1 -> Equal6/2
  Constant5/1 -> Equal7/2
  Equal6/1 -> Logical Operator1/1
  Equal7/1 -> Logical Operator1/2
  Logical Operator1/1 -> Logical Operator30/6
  [VINP_FrEDUDrtStaNidec_flg] -> Equal10/1
  Constant6/1 -> Equal10/2
  Equal10/1 -> Logical Operator30/7
  Equal2/1 -> Logical Operator30/8
  [VDDM_MCUNF1CSErrCFS_flg] -> Logical Operator10/1
  [VDDM_MCUNF1RCErrCFS_flg] -> Logical Operator9/1
  Logical Operator9/1 -> Logical Operator30/4
  [VDDM_MCUNF1NoComCFS_flg] -> Logical Operator7/1
  Logical Operator7/1 -> Logical Operator30/3
  Logical Operator10/1 -> Logical Operator30/5
  [VDDM_MCUNR1CSErrCFS_flg] -> Logical Operator17/1
  Equal33/1 -> Logical Operator16/1
  [VINP_MCUWarnRNidec_enum] -> Equal33/1
  [VINP_VehSpeed_kph] -> Equal23/1
  [VINP_MCUWarnRNidec_enum] -> Equal34/1
  Logical Operator17/1 -> Logical Operator27/5
  Equal34/1 -> Logical Operator16/2
  [VDDM_MCUNR1NoComCFS_flg] -> Logical Operator35/1
  Constant33/1 -> Equal24/2
  Equal23/1 -> Logical Operator27/8
  Equal9/1 -> Logical Operator27/7
  [VDDM_MCUNR1RCErrCFS_flg] -> Logical Operator37/1
  Constant35/1 -> Equal9/2
  Logical Operator35/1 -> Logical Operator27/3
  Constant32/1 -> Equal33/2
  [VINP_RrEDUDrtStaNidec_flg] -> Equal9/1
  Constant34/1 -> Equal34/2
  [No_CAN_BUS_OFF] -> Logical Operator27/2
  Constant31/1 -> Equal23/2
  Logical Operator16/1 -> Logical Operator27/6
  Equal24/1 -> Logical Operator27/1
  [VPMM_SysPwrSta_enum] -> Equal24/1
  Logical Operator37/1 -> Logical Operator27/4
  Logical Operator11/1 -> Logical Operator34/1, Timer1/1
  [task_time_s] -> Test Detection Criteria1/2
  [task_time_s] -> Timer1/3
  Constant42/1 -> Switch6/1
  Test Detection Criteria1/1 -> [VDDM_FrMCUNTqErrDet_flg]  "VDDM_FrMCUNTqErrDet_flg"
  Logical Operator34/1 -> Timer1/2
  Timer1/1 -> Equal27/1
  Constant43/1 -> Test Detection Criteria1/3
  Switch6/1 -> Test Detection Criteria1/1
  Equal27/1 -> [VDDM_FrMCUNTqErrPass_flg]  "VDDM_FrMCUNTqErrPass_flg"
  Logical Operator30/1 -> Switch6/3
  Constant46/1 -> Test Detection Criteria1/4
  Constant70/1 -> Timer1/4
  Constant45/1 -> Equal27/2
  [VDDM_FrMCUNTqErrCFSRls_flg] -> Switch6/2
  [VDDM_FrMCUNTqErrDet_flg] -> DTC_Info/1
  DTC_Info/1 -> VDDM_FrMCUTqErrDTC_raw32/1  "VDDM_FrMCUTqErrDTC_raw32"
  [DTC_clear_request] -> DTC_Info/4
  [VDDM_FrMCUNTqErrCFS_flg] -> DTC_Info/3
  [VDDM_FrMCUNTqErrPass_flg] -> DTC_Info/2
  [VDDM_RrMCUNTqErrCFSRls_flg] -> Switch1/2
  Test Detection Criteria2/1 -> [VDDM_RrMCUNTqErrDet_flg]  "VDDM_RrMCUNTqErrDet_flg"
  [VDDM_RrMCUNTqErrDet_flg] -> DTC_Info1/1
  DTC_Info1/1 -> VDDM_RrMCUTqErrDTC_raw32/1  "VDDM_RrMCUTqErrDTC_raw32"
  [DTC_clear_request] -> DTC_Info1/4
  Equal5/1 -> [VDDM_RrMCUNTqErrPass_flg]  "VDDM_RrMCUNTqErrPass_flg"
  [VDDM_RrMCUNTqErrCFS_flg] -> DTC_Info1/3
  Constant39/1 -> Timer2/4
  Constant24/1 -> Switch1/1
  [task_time_s] -> Timer2/3
  Timer2/1 -> Equal5/1
  [VDDM_RrMCUNTqErrPass_flg] -> DTC_Info1/2
  [task_time_s] -> Test Detection Criteria2/2
  Constant28/1 -> Test Detection Criteria2/3
  Logical Operator27/1 -> Switch1/3
  Constant37/1 -> Test Detection Criteria2/4
  Switch1/1 -> Test Detection Criteria2/1
  Logical Operator28/1 -> Timer2/2
  Constant36/1 -> Equal5/2
  Logical Operator6/1 -> Logical Operator28/1, Timer2/1
  task_time_s/1 -> [task_time_s]
  VPMM_SysPwrSta_enum/1 -> [VPMM_SysPwrSta_enum]
  No_CAN3_BUS_OFF/1 -> [No_CAN_BUS_OFF]
  VDDM_MCUNF1NoComCFS_flg/1 -> [VDDM_MCUNF1NoComCFS_flg]
  VDDM_MCUNF1RCErrCFS_flg/1 -> [VDDM_MCUNF1RCErrCFS_flg]
  VDDM_MCUNF1CSErrCFS_flg/1 -> [VDDM_MCUNF1CSErrCFS_flg]
  VINP_FrEDUDrtStaNidec_flg/1 -> [VINP_FrEDUDrtStaNidec_flg]
  VINP_VehSpeed_kph/1 -> [VINP_VehSpeed_kph]
  VTQR_FrTMTqReq_Nm/1 -> Round1/1
  VDDM_MCUNR1NoComCFS_flg/1 -> [VDDM_MCUNR1NoComCFS_flg]
  VDDM_MCUNR1RCErrCFS_flg/1 -> [VDDM_MCUNR1RCErrCFS_flg]
  VDDM_MCUNR1CSErrCFS_flg/1 -> [VDDM_MCUNR1CSErrCFS_flg]
  VINP_RrEDUDrtStaNidec_flg/1 -> [VINP_RrEDUDrtStaNidec_flg]
  VTQR_RrTMTqReq_Nm/1 -> Round/1
  DTC_clear_request/1 -> [DTC_clear_request]
  [VINP_MCUWarnFNidec_enum] -> Equal6/1
  [VINP_MCUWarnFNidec_enum] -> Equal7/1
  Round/1 -> [VTQR_RrTMTqReq_Nm]
  VINP_RrEDURealTMTqNidec_Nm/1 -> [VINP_RrEDURealTMTqNidec_Nm]
  Round1/1 -> [VTQR_FrTMTqReq_Nm]
  VINP_FrEDURealTMTqNidec_Nm/1 -> [VINP_FrEDURealTMTqNidec_Nm]
  OR/1 -> Logical Operator30/10
  Constant15/1 -> Equal/2
  Constant49/1 -> Equal25/2
  [VPMM_DrivetrainSelect_enum] -> Equal25/1
  [VPMM_DrivetrainSelect_enum] -> Equal/1
  Equal25/1 -> OR/2
  Equal/1 -> OR/1
  [VTQR_FrTMTqReq_Nm] -> Abs4/1
  MDDM_FrTMTqDev_Y_Nm/1 -> [VDDM_FrTMTqDev_Nm], Equal12/2  "VDDM_FrTMTqDev_Nm"
  Abs/1 -> Equal12/1  "VDDM_FrTMTqDiffAbs_Nm"
  Add/1 -> Abs/1
  [VINP_FrEDURealTMTqNidec_Nm] -> Add/1
  Equal12/1 -> Logical Operator30/9  "VDDM_FrTMTqDiffGTDev_flg"
  Abs4/1 -> MDDM_FrTMTqDev_Y_Nm/1
  [VTQR_FrTMTqReq_Nm] -> Add/2
  VPMM_DrivetrainSelect_enum/1 -> [VPMM_DrivetrainSelect_enum]
  [VPMM_DrivetrainSelect_enum] -> Equal1/1
  Equal15/1 -> OR1/2
  Constant1/1 -> Equal1/2
  Add1/1 -> Abs1/1
  [No_CAN_BUS_OFF] -> Logical Operator11/2
  Equal14/1 -> Logical Operator11/8
  Equal11/1 -> Logical Operator11/7
  Equal28/1 -> Logical Operator2/1
  Logical Operator14/1 -> Logical Operator11/4
  Logical Operator3/1 -> Logical Operator11/5
  Logical Operator2/1 -> Logical Operator11/6
  [VINP_VehSpeed_kph] -> Equal14/1
  Equal1/1 -> OR1/1
  Constant7/1 -> Equal14/2
  [VPMM_SysPwrSta_enum] -> Equal16/1
  Constant21/1 -> Equal29/2
  Constant17/1 -> Equal16/2
  Constant20/1 -> Equal15/2
  [VPMM_DrivetrainSelect_enum] -> Equal15/1
  Equal16/1 -> Logical Operator11/1
  Logical Operator13/1 -> Logical Operator11/3
  Constant41/1 -> Equal11/2
  [VDDM_MCUNF1NoComCFS_flg] -> Logical Operator13/1
  [VDDM_MCUNF1RCErrCFS_flg] -> Logical Operator14/1
  [VINP_MCUWarnFNidec_enum] -> Equal29/1
  [VINP_FrEDUDrtStaNidec_flg] -> Equal11/1
  Constant16/1 -> Equal28/2
  Abs1/1 -> Equal13/1
  [VINP_MCUWarnFNidec_enum] -> Equal28/1
  Equal29/1 -> Logical Operator2/2
  [VINP_FrEDURealTMTqNidec_Nm] -> Add1/1
  [VTQR_FrTMTqReq_Nm] -> Add1/2
  OR1/1 -> Logical Operator11/10
  [VDDM_MCUNF1CSErrCFS_flg] -> Logical Operator3/1
  Equal13/1 -> Logical Operator15/1
  Logical Operator15/1 -> Logical Operator11/9
  Constant52/1 -> Relational Operator2/2
  [VDDM_FrMCUNTqErrDet_flg] -> DTC_Couter3/1
  DTC_Couter3/2 -> Relational Operator2/1  "VDDM_FrMCUNTqErrDTC_cnt"
  [VDDM_FrMCUNTqErrCFSRls_flg] -> DTC_Couter3/2
  Logical Operator41/1 -> [VDDM_FrMCUNTqErrCFSRls_flg]  "VDDM_FrMCUNTqErrCFSRls_flg"
  DTC_Couter3/1 -> [VDDM_FrMCUNTqErrCFS_flg]  "VDDM_FrMCUNTqErrCFS_flg"
  Constant54/1 -> DTC_Couter3/3
  Logical Operator43/1 -> Logical Operator41/3
  [VDDM_FrMCUNTqErrPass_flg] -> Logical Operator43/1
  Relational Operator2/1 -> Terminator/1  "VDDM_FrMCUNTqErrDFS_flg"
  Logical Operator20/1 -> Logical Operator41/1
  NOT1/1 -> Logical Operator43/2
  [DTC_clear_request] -> Logical Operator41/2
  Constant51/1 -> Logical Operator41/4
  [VDDM_FrMCUNTqErrCFS_flg] -> Delay1/1
  Delay1/1 -> NOT1/1
  [VTQR_RrTMTqReq_Nm] -> Abs6/1
  Abs2/1 -> Equal18/1  "VDDM_RrTMTqDiffAbs_Nm"
  Abs6/1 -> MDDM_RrTMTqDev_Y_Nm/1
  OR2/1 -> Logical Operator27/10
  [VPMM_DrivetrainSelect_enum] -> Equal3/1
  Constant8/1 -> Equal4/2
  Constant2/1 -> Equal3/2
  Equal3/1 -> OR2/1
  Equal4/1 -> OR2/2
  Add2/1 -> Abs2/1
  Equal18/1 -> Logical Operator27/9  "VDDM_RrTMTqDiffGTDev_flg"
  [VTQR_RrTMTqReq_Nm] -> Add2/2
  [VPMM_DrivetrainSelect_enum] -> Equal4/1
  [VINP_RrEDURealTMTqNidec_Nm] -> Add2/1
  MDDM_RrTMTqDev_Y_Nm/1 -> [VDDM_RrTMTqDev_Nm], Equal18/2  "VDDM_RrTMTqDev_Nm"
  Add3/1 -> Abs3/1
  [VPMM_DrivetrainSelect_enum] -> Equal20/1
  Logical Operator4/1 -> Logical Operator6/6
  Logical Operator12/1 -> Logical Operator6/4
  [No_CAN_BUS_OFF] -> Logical Operator6/2
  Constant14/1 -> Equal22/2
  Logical Operator8/1 -> Logical Operator6/3
  Constant25/1 -> Equal37/2
  [VDDM_MCUNR1NoComCFS_flg] -> Logical Operator8/1
  Equal37/1 -> Logical Operator6/7
  Constant13/1 -> Equal19/2
  Equal22/1 -> Logical Operator4/2
  Equal21/1 -> Logical Operator4/1
  [VDDM_MCUNR1CSErrCFS_flg] -> Logical Operator5/1
  [VINP_RrEDURealTMTqNidec_Nm] -> Add3/1
  Equal19/1 -> Logical Operator6/1
  [VPMM_SysPwrSta_enum] -> Equal19/1
  [VINP_VehSpeed_kph] -> Equal17/1
  [VINP_MCUWarnRNidec_enum] -> Equal22/1
  Logical Operator5/1 -> Logical Operator6/5
  Constant10/1 -> Equal17/2
  [VINP_MCUWarnRNidec_enum] -> Equal21/1
  Abs3/1 -> Equal8/1
  Equal36/1 -> OR3/2
  [VPMM_DrivetrainSelect_enum] -> Equal36/1
  [VINP_RrEDUDrtStaNidec_flg] -> Equal37/1
  Equal20/1 -> OR3/1
  [VDDM_MCUNR1RCErrCFS_flg] -> Logical Operator12/1
  OR3/1 -> Logical Operator6/10
  [VTQR_RrTMTqReq_Nm] -> Add3/2
  Constant9/1 -> Equal20/2
  Equal17/1 -> Logical Operator6/8
  Constant11/1 -> Equal21/2
  Constant26/1 -> Equal36/2
  Equal8/1 -> Logical Operator18/1
  Logical Operator18/1 -> Logical Operator6/9
  Constant30/1 -> Relational Operator1/2
  DTC_Couter1/2 -> Relational Operator1/1  "VDDM_RrMCUNTqErrDTC_cnt"
  [DTC_clear_request] -> Logical Operator19/2
  Constant18/1 -> DTC_Couter1/3
  Constant29/1 -> Logical Operator19/4
  NOT2/1 -> Logical Operator22/2
  Delay2/1 -> NOT2/1
  [VDDM_RrMCUNTqErrCFSRls_flg] -> DTC_Couter1/2
  DTC_Couter1/1 -> [VDDM_RrMCUNTqErrCFS_flg]  "VDDM_RrMCUNTqErrCFS_flg"
  Logical Operator21/1 -> Logical Operator19/1
  [VDDM_RrMCUNTqErrDet_flg] -> DTC_Couter1/1
  [VDDM_RrMCUNTqErrCFS_flg] -> Delay2/1
  Relational Operator1/1 -> Terminator1/1  "VDDM_RrMCUNTqErrDFS_flg"
  [VDDM_RrMCUNTqErrPass_flg] -> Logical Operator22/1
  Logical Operator22/1 -> Logical Operator19/3
  Logical Operator19/1 -> [VDDM_RrMCUNTqErrCFSRls_flg]  "VDDM_RrMCUNTqErrCFSRls_flg"
  [VDDM_FrTMTqDev_Nm] -> Equal13/2
  [VDDM_RrTMTqDev_Nm] -> Equal8/2
  [VDDM_FrMCUNTqErrCFS_flg] -> VDDM_FrMCUNTqErrCFS_flg/1
  [VDDM_RrMCUNTqErrCFS_flg] -> VDDM_RrMCUNTqErrCFS_flg/1
  Constant19/1 -> Equal31/2
  Constant12/1 -> Equal30/2
  [VPMM_SysPwrSta_enum] -> Equal30/1
  Equal31/1 -> Logical Operator20/1
  Unit Delay5/1 -> Equal31/1
  Equal30/1 -> Logical Operator20/2
  [VPMM_SysPwrSta_enum] -> Unit Delay5/1
  Constant23/1 -> Equal35/2
  Constant22/1 -> Equal32/2
  [VPMM_SysPwrSta_enum] -> Equal32/1
  Equal35/1 -> Logical Operator21/1
  Unit Delay1/1 -> Equal35/1
  Equal32/1 -> Logical Operator21/2
  [VPMM_SysPwrSta_enum] -> Unit Delay1/1
  VINP_MCUWarnFNidec_enum/1 -> [VINP_MCUWarnFNidec_enum]
  VINP_MCUWarnRNidec_enum/1 -> [VINP_MCUWarnRNidec_enum]
